simulink model "gm_parallel_8_phase_voltages"  (R2022a)
settings: Solver=FixedStepDiscrete  StartTime=0.0  StopTime=10.0  RelTol=1e-3
undefined symbols (not defined in the file or in its folder): f_c, u_dc
libraries: hdlmdlgenlib x14, simulink x2
(part 2 of 4)

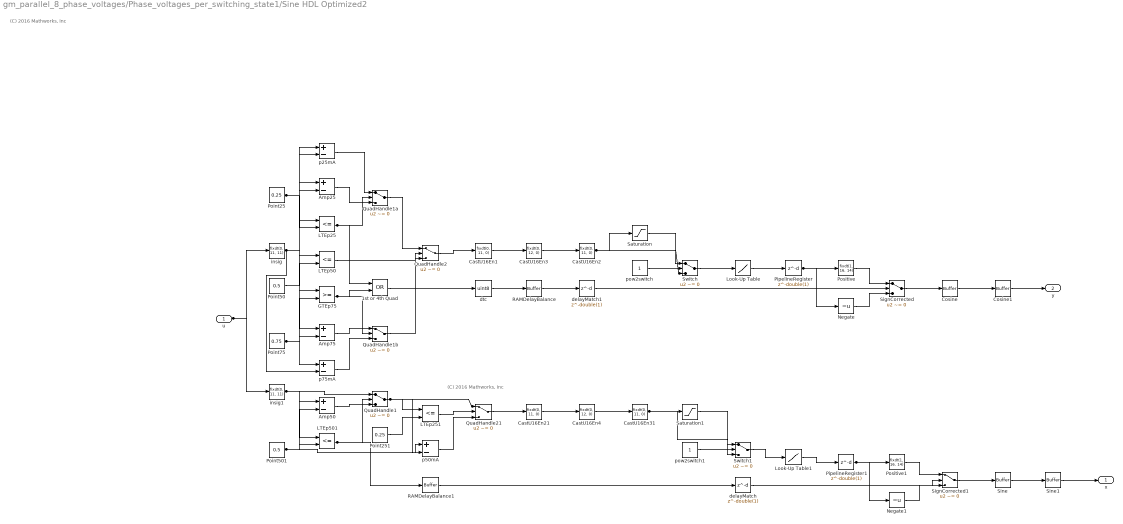
== system gm_parallel_8_phase_voltages/Phase_voltages_per_switching_state1/Sine HDL Optimized2 ==
  note: (C) 2016 Mathworks, Inc
  note: (C) 2016 Mathworks, Inc
  u : Inport  OutDataTypeStr=fixdt(1,24,20,'DataTypeOverride', 'Off')  SampleTime=1e-08
  1st or 4th Quad : Logic  Operator=OR  AllPortsSameDT=off  OutDataTypeStr=boolean  SampleTime=1e-08
  Amp25 : Sum  Inputs=+-  AccumDataTypeStr=fixdt(1, 17, 16)  OutDataTypeStr=fixdt(1, 17, 16)  SampleTime=1e-08
  Amp50 : Sum  Inputs=+-  AccumDataTypeStr=fixdt(1, 17, 16)  OutDataTypeStr=fixdt(1, 17, 16)  SampleTime=1e-08
  Amp75 : Sum  Inputs=+-  AccumDataTypeStr=fixdt(1, 17, 16)  OutDataTypeStr=fixdt(1, 17, 16)  SampleTime=1e-08
  CastU16En1 : DataTypeConversion  OutDataTypeStr=fixdt(0, 11, 0)  ConvertRealWorld=Stored Integer (SI)  SampleTime=1e-08  SaturateOnIntegerOverflow=off  RndMeth=Floor
  CastU16En2 : DataTypeConversion  OutDataTypeStr=fixdt(0, 11, 0)  ConvertRealWorld=Stored Integer (SI)  SampleTime=1e-08  RndMeth=Floor
  CastU16En21 : DataTypeConversion  OutDataTypeStr=fixdt(0, 11, 0)  ConvertRealWorld=Stored Integer (SI)  SampleTime=1e-08  SaturateOnIntegerOverflow=off  RndMeth=Floor
  CastU16En3 : DataTypeConversion  OutDataTypeStr=fixdt(0, 12, 0)  SampleTime=1e-08  SaturateOnIntegerOverflow=off  RndMeth=Floor
  CastU16En31 : DataTypeConversion  OutDataTypeStr=fixdt(0, 11, 0)  ConvertRealWorld=Stored Integer (SI)  SampleTime=1e-08  RndMeth=Floor
  CastU16En4 : DataTypeConversion  OutDataTypeStr=fixdt(0, 12, 0)  SampleTime=1e-08  SaturateOnIntegerOverflow=off  RndMeth=Floor
  Cosine : hdlmdlgenlib/Buffer
      settings: SourceProductBaseCode=SL
  Cosine1 : hdlmdlgenlib/Buffer
      settings: SourceProductBaseCode=SL
  GTEp75 : RelationalOperator  OutDataTypeStr=boolean  SampleTime=1e-08  InputSameDT=off
  LTEp{25,50,251,501} (4 alike) : RelationalOperator  Operator=<=  OutDataTypeStr=boolean  SampleTime=1e-08  InputSameDT=off
  Look-Up Table : Lookup_n-D  NumberOfTableDimensions=1  BreakpointsForDimension1="fi(\"numerictype\",numerictype(0,11,0),\"fimath\",fimath(\"RoundingMethod\", \"Floor\",\"OverflowAction\", \"Wrap\",\"ProductMode\",\"FullPrecision\",\"SumMode\",\"FullPrecision\"),\"Value\",\"[0 1 2 3 4 5 6 7 8 9 10 11 12 13 14 15 16 17 18 19 20 21 22 23 24 25 26 27 28 29 30 31 32 33 34 35 36 37 38 39 40 41 42 43 44 45 46 47 48 49 50 51 52 53 54 55 56 57 58 59 60 61 62 63 64 65 66 67 68 69 70 71 72 73 74 75 76 77 78 79 80 81 82 83 84 85 86 87 88 89 90 91 92 93 94 95 96 97 98 99 100 101 102 103 104 105 106 107 108 109 110 111 112 113 114 115 116 117 118 119 120 121 122 123 124 125 126 127 128 129 130 131 132 133 134 135 136 137 138 139 140 141 142 143 144 145 146 147 148 149 150 151 152 153 154 155 156 157 158 159 160 161 162 163 164 165 166 167 168 169 170 171 172 173 174 175 176 177 178 179 180 181 182 183 184 185 186 187 188 189 190 191 192 193 194 195 196 197 198 199 200 201 202 203 204 205 206 207 208 209 210 211 212 213 214 215 216 217 218 219 220 221 222 223 224 225 226 227 228 229 230 231 232 233 234 235 236 237 238 239 240 241 242 243 244 245 246 247 248 249 250 251 252 253 254 255 256 257 258 259 260 261 262 263 264 265 266 267 268 269 270 271 272 273 274 275 276 277 278 279 280 281 282 283 284 285 286 287 288 289 290 291 292 293 294 295 296 297 298 299 300 301 302 303 304 305 306 307 308 309 310 311 312 313 314 315 316 317 318 319 320 321 322 323 324 325 326 327 328 329 330 331 332 333 334 335 336 337 338 339 340 341 342 343 344 345 346 347 348 349 350 351 352 353 354 355 356 357 358 359 360 361 362 363 364 365 366 367 368 369 370 371 372 373 374 375 376 377 378 379 380 381 382 383 384 385 386 387 388 389 390 391 392 393 394 395 396 397 398 399 400 401 402 403 404 405 406 407 408 409 410 411 412 413 414 415 416 417 418 419 420 421 422 423 424 425 426 427 428 429 430 431 432 433 434 435 436 437 438 439 440 441 442 443 444 445 446 447 448 449 450 451 452 453 454 455 456 457 458 459 460 461 462 463 464 465 466 467 468 469 470 471 472 473 474 475 476 477 478 479 480 481 482 483 484 485 486 487 488 489 490 491 492 493 494 495 496 497 498 499 500 501 502 503 504 505 506 507 508 509 510 511]\")"  Table="reshape(fi(\"numerictype\",numerictype(1,16,14),\"fimath\",fimath(\"RoundingMethod\", \"Floor\",\"OverflowAction\", \"Wrap\",\"ProductMode\",\"FullPrecision\",\"SumMode\",\"FullPrecision\"),\"Value\",\"[0;0.0030517578125;0.00616455078125;0.00921630859375;0.01226806640625;0.015380859375;0.0184326171875;0.02154541015625;0.02459716796875;0.02764892578125;0.03076171875;0.0338134765625;0.036865234375;0.03997802734375;0.04302978515625;0.04608154296875;0.04913330078125;0.05224609375;0.0552978515625;0.058349609375;0.06146240234375;0.06451416015625;0.06756591796875;0.07061767578125;0.07373046875;0.0767822265625;0.079833984375;0.0828857421875;0.0859375;0.08905029296875;0.09210205078125;0.09515380859375;0.09820556640625;0.10125732421875;0.10430908203125;0.10736083984375;0.11041259765625;0.11346435546875;0.11651611328125;0.11956787109375;0.12261962890625;0.12567138671875;0.12872314453125;0.13177490234375;0.13482666015625;0.13787841796875;0.14093017578125;0.14398193359375;0.14703369140625;0.15008544921875;0.153076171875;0.1561279296875;0.1591796875;0.16217041015625;0.16522216796875;0.16827392578125;0.1712646484375;0.17431640625;0.1773681640625;0.18035888671875;0.18341064453125;0.1864013671875;0.189453125;0.19244384765625;0.19549560546875;0.198486328125;0.20147705078125;0.20452880859375;0.20751953125;0.21051025390625;0.2135009765625;0.216552734375;0.21954345703125;0.2225341796875;0.22552490234375;0.228515625;0.23150634765625;0.2344970703125;0.23748779296875;0.240478515625;0.24346923828125;0.24639892578125;0.2493896484375;0.25238037109375;0.25537109375;0.25830078125;0.26129150390625;0.2642822265625;0.2672119140625;0.27020263671875;0.27313232421875;0.276123046875;0.279052734375;0.281982421875;0.28497314453125;0.28790283203125;0.29083251953125;0.29376220703125;0.29669189453125;0.29962158203125;0.30255126953125;0.30548095703125;0.30841064453125;0.31134033203125;0.31427001953125;0.31719970703125;0.32012939453125;0.322998046875;0.325927734375;0.328857421875;0.33172607421875;0.33465576171875;0.3375244140625;0.34039306640625;0.34332275390625;0.34619140625;0.34906005859375;0.3519287109375;0.35479736328125;0.35772705078125;0.360595703125;0.3634033203125;0.36627197265625;0.369140625;0.37200927734375;0.3748779296875;0.377685546875;0.38055419921875;0.3834228515625;0.38623046875;0.3890380859375;0.39190673828125;0.39471435546875;0.39752197265625;0.400390625;0.4031982421875;0.406005859375;0.4088134765625;0.41162109375;0.41436767578125;0.41717529296875;0.41998291015625;0.42279052734375;0.425537109375;0.4283447265625;0.43109130859375;0.43389892578125;0.4366455078125;0.43939208984375;0.44219970703125;0.4449462890625;0.44769287109375;0.450439453125;0.45318603515625;0.4559326171875;0.4586181640625;0.46136474609375;0.464111328125;0.466796875;0.46954345703125;0.47222900390625;0.4749755859375;0.4776611328125;0.4803466796875;0.4830322265625;0.4857177734375;0.4884033203125;0.4910888671875;0.4937744140625;0.4964599609375;0.49908447265625;0.50177001953125;0.50445556640625;0.507080078125;0.50970458984375;0.51239013671875;0.5150146484375;0.51763916015625;0.520263671875;0.52288818359375;0.5255126953125;0.52813720703125;0.53070068359375;0.5333251953125;0.53594970703125;0.53851318359375;0.5411376953125;0.543701171875;0.5462646484375;0.548828125;0.5513916015625;0.553955078125;0.5565185546875;0.55908203125;0.5616455078125;0.56414794921875;0.56671142578125;0.5692138671875;0.57177734375;0.57427978515625;0.5767822265625;0.57928466796875;0.581787109375;0.58428955078125;0.5867919921875;0.58929443359375;0.59173583984375;0.59423828125;0.5966796875;0.59918212890625;0.60162353515625;0.60406494140625;0.60650634765625;0.60894775390625;0.61138916015625;0.61383056640625;0.61627197265625;0.61865234375;0.62109375;0.62347412109375;0.62591552734375;0.6282958984375;0.63067626953125;0.633056640625;0.63543701171875;0.6378173828125;0.64019775390625;0.64251708984375;0.6448974609375;0.647216796875;0.6495361328125;0.65191650390625;0.65423583984375;0.65655517578125;0.65887451171875;0.66119384765625;0.6634521484375;0.665771484375;0.6680908203125;0.67034912109375;0.672607421875;0.6749267578125;0.67718505859375;0.679443359375;0.68170166015625;0.68389892578125;0.6861572265625;0.68841552734375 ...(+4183 chars)]\"), [1  512])"  InterpMethod=Flat  ExtrapMethod=Clip  DiagnosticForOutOfRangeInput=Error  SampleTime=1e-08  OutDataTypeStr=fixdt(1, 16, 14)
  Look-Up Table1 : Lookup_n-D  NumberOfTableDimensions=1  BreakpointsForDimension1="fi(\"numerictype\",numerictype(0,11,0),\"fimath\",fimath(\"RoundingMethod\", \"Floor\",\"OverflowAction\", \"Wrap\",\"ProductMode\",\"FullPrecision\",\"SumMode\",\"FullPrecision\"),\"Value\",\"[0 1 2 3 4 5 6 7 8 9 10 11 12 13 14 15 16 17 18 19 20 21 22 23 24 25 26 27 28 29 30 31 32 33 34 35 36 37 38 39 40 41 42 43 44 45 46 47 48 49 50 51 52 53 54 55 56 57 58 59 60 61 62 63 64 65 66 67 68 69 70 71 72 73 74 75 76 77 78 79 80 81 82 83 84 85 86 87 88 89 90 91 92 93 94 95 96 97 98 99 100 101 102 103 104 105 106 107 108 109 110 111 112 113 114 115 116 117 118 119 120 121 122 123 124 125 126 127 128 129 130 131 132 133 134 135 136 137 138 139 140 141 142 143 144 145 146 147 148 149 150 151 152 153 154 155 156 157 158 159 160 161 162 163 164 165 166 167 168 169 170 171 172 173 174 175 176 177 178 179 180 181 182 183 184 185 186 187 188 189 190 191 192 193 194 195 196 197 198 199 200 201 202 203 204 205 206 207 208 209 210 211 212 213 214 215 216 217 218 219 220 221 222 223 224 225 226 227 228 229 230 231 232 233 234 235 236 237 238 239 240 241 242 243 244 245 246 247 248 249 250 251 252 253 254 255 256 257 258 259 260 261 262 263 264 265 266 267 268 269 270 271 272 273 274 275 276 277 278 279 280 281 282 283 284 285 286 287 288 289 290 291 292 293 294 295 296 297 298 299 300 301 302 303 304 305 306 307 308 309 310 311 312 313 314 315 316 317 318 319 320 321 322 323 324 325 326 327 328 329 330 331 332 333 334 335 336 337 338 339 340 341 342 343 344 345 346 347 348 349 350 351 352 353 354 355 356 357 358 359 360 361 362 363 364 365 366 367 368 369 370 371 372 373 374 375 376 377 378 379 380 381 382 383 384 385 386 387 388 389 390 391 392 393 394 395 396 397 398 399 400 401 402 403 404 405 406 407 408 409 410 411 412 413 414 415 416 417 418 419 420 421 422 423 424 425 426 427 428 429 430 431 432 433 434 435 436 437 438 439 440 441 442 443 444 445 446 447 448 449 450 451 452 453 454 455 456 457 458 459 460 461 462 463 464 465 466 467 468 469 470 471 472 473 474 475 476 477 478 479 480 481 482 483 484 485 486 487 488 489 490 491 492 493 494 495 496 497 498 499 500 501 502 503 504 505 506 507 508 509 510 511]\")"  Table="reshape(fi(\"numerictype\",numerictype(1,16,14),\"fimath\",fimath(\"RoundingMethod\", \"Floor\",\"OverflowAction\", \"Wrap\",\"ProductMode\",\"FullPrecision\",\"SumMode\",\"FullPrecision\"),\"Value\",\"[0;0.0030517578125;0.00616455078125;0.00921630859375;0.01226806640625;0.015380859375;0.0184326171875;0.02154541015625;0.02459716796875;0.02764892578125;0.03076171875;0.0338134765625;0.036865234375;0.03997802734375;0.04302978515625;0.04608154296875;0.04913330078125;0.05224609375;0.0552978515625;0.058349609375;0.06146240234375;0.06451416015625;0.06756591796875;0.07061767578125;0.07373046875;0.0767822265625;0.079833984375;0.0828857421875;0.0859375;0.08905029296875;0.09210205078125;0.09515380859375;0.09820556640625;0.10125732421875;0.10430908203125;0.10736083984375;0.11041259765625;0.11346435546875;0.11651611328125;0.11956787109375;0.12261962890625;0.12567138671875;0.12872314453125;0.13177490234375;0.13482666015625;0.13787841796875;0.14093017578125;0.14398193359375;0.14703369140625;0.15008544921875;0.153076171875;0.1561279296875;0.1591796875;0.16217041015625;0.16522216796875;0.16827392578125;0.1712646484375;0.17431640625;0.1773681640625;0.18035888671875;0.18341064453125;0.1864013671875;0.189453125;0.19244384765625;0.19549560546875;0.198486328125;0.20147705078125;0.20452880859375;0.20751953125;0.21051025390625;0.2135009765625;0.216552734375;0.21954345703125;0.2225341796875;0.22552490234375;0.228515625;0.23150634765625;0.2344970703125;0.23748779296875;0.240478515625;0.24346923828125;0.24639892578125;0.2493896484375;0.25238037109375;0.25537109375;0.25830078125;0.26129150390625;0.2642822265625;0.2672119140625;0.27020263671875;0.27313232421875;0.276123046875;0.279052734375;0.281982421875;0.28497314453125;0.28790283203125;0.29083251953125;0.29376220703125;0.29669189453125;0.29962158203125;0.30255126953125;0.30548095703125;0.30841064453125;0.31134033203125;0.31427001953125;0.31719970703125;0.32012939453125;0.322998046875;0.325927734375;0.328857421875;0.33172607421875;0.33465576171875;0.3375244140625;0.34039306640625;0.34332275390625;0.34619140625;0.34906005859375;0.3519287109375;0.35479736328125;0.35772705078125;0.360595703125;0.3634033203125;0.36627197265625;0.369140625;0.37200927734375;0.3748779296875;0.377685546875;0.38055419921875;0.3834228515625;0.38623046875;0.3890380859375;0.39190673828125;0.39471435546875;0.39752197265625;0.400390625;0.4031982421875;0.406005859375;0.4088134765625;0.41162109375;0.41436767578125;0.41717529296875;0.41998291015625;0.42279052734375;0.425537109375;0.4283447265625;0.43109130859375;0.43389892578125;0.4366455078125;0.43939208984375;0.44219970703125;0.4449462890625;0.44769287109375;0.450439453125;0.45318603515625;0.4559326171875;0.4586181640625;0.46136474609375;0.464111328125;0.466796875;0.46954345703125;0.47222900390625;0.4749755859375;0.4776611328125;0.4803466796875;0.4830322265625;0.4857177734375;0.4884033203125;0.4910888671875;0.4937744140625;0.4964599609375;0.49908447265625;0.50177001953125;0.50445556640625;0.507080078125;0.50970458984375;0.51239013671875;0.5150146484375;0.51763916015625;0.520263671875;0.52288818359375;0.5255126953125;0.52813720703125;0.53070068359375;0.5333251953125;0.53594970703125;0.53851318359375;0.5411376953125;0.543701171875;0.5462646484375;0.548828125;0.5513916015625;0.553955078125;0.5565185546875;0.55908203125;0.5616455078125;0.56414794921875;0.56671142578125;0.5692138671875;0.57177734375;0.57427978515625;0.5767822265625;0.57928466796875;0.581787109375;0.58428955078125;0.5867919921875;0.58929443359375;0.59173583984375;0.59423828125;0.5966796875;0.59918212890625;0.60162353515625;0.60406494140625;0.60650634765625;0.60894775390625;0.61138916015625;0.61383056640625;0.61627197265625;0.61865234375;0.62109375;0.62347412109375;0.62591552734375;0.6282958984375;0.63067626953125;0.633056640625;0.63543701171875;0.6378173828125;0.64019775390625;0.64251708984375;0.6448974609375;0.647216796875;0.6495361328125;0.65191650390625;0.65423583984375;0.65655517578125;0.65887451171875;0.66119384765625;0.6634521484375;0.665771484375;0.6680908203125;0.67034912109375;0.672607421875;0.6749267578125;0.67718505859375;0.679443359375;0.68170166015625;0.68389892578125;0.6861572265625;0.68841552734375 ...(+4183 chars)]\"), [1  512])"  InterpMethod=Flat  ExtrapMethod=Clip  DiagnosticForOutOfRangeInput=Error  SampleTime=1e-08  OutDataTypeStr=fixdt(1, 16, 14)
  Negate : UnaryMinus  SampleTime=1e-08
  Negate1 : UnaryMinus  SampleTime=1e-08
  PipelineRegister : Delay  DelayLength=double(1)  InitialCondition=0  SampleTime=1e-08
  PipelineRegister1 : Delay  DelayLength=double(1)  InitialCondition=0  SampleTime=1e-08
  Point25 : Constant  Value=0.25  OutDataTypeStr=fixdt(0, 16, 16)  SampleTime=1e-08
  Point251 : Constant  Value=0.25  OutDataTypeStr=fixdt(0, 16, 16)  SampleTime=1e-08
  Point50 : Constant  Value=0.5  OutDataTypeStr=fixdt(0, 16, 16)  SampleTime=1e-08
  Point501 : Constant  Value=0.5  OutDataTypeStr=fixdt(0, 16, 16)  SampleTime=1e-08
  Point75 : Constant  Value=0.75  OutDataTypeStr=fixdt(0, 16, 16)  SampleTime=1e-08
  Positive : DataTypeConversion  OutDataTypeStr=fixdt(1, 16, 14)  SampleTime=1e-08  SaturateOnIntegerOverflow=off  RndMeth=Floor
  Positive1 : DataTypeConversion  OutDataTypeStr=fixdt(1, 16, 14)  SampleTime=1e-08  SaturateOnIntegerOverflow=off  RndMeth=Floor
  QuadHandle1 : Switch  Criteria=u2 ~= 0  Threshold=double(0)  OutDataTypeStr=fixdt(1, 17, 16)  SampleTime=1e-08  SaturateOnIntegerOverflow=off  InputSameDT=off
  QuadHandle1a : Switch  Criteria=u2 ~= 0  Threshold=double(0)  OutDataTypeStr=fixdt(1, 17, 16)  SampleTime=1e-08  SaturateOnIntegerOverflow=off  InputSameDT=off
  QuadHandle1b : Switch  Criteria=u2 ~= 0  Threshold=double(0)  OutDataTypeStr=fixdt(1, 17, 16)  SampleTime=1e-08  SaturateOnIntegerOverflow=off  InputSameDT=off
  QuadHandle2 : Switch  Criteria=u2 ~= 0  Threshold=double(0)  OutDataTypeStr=fixdt(0, 11, 11)  SampleTime=1e-08  InputSameDT=off
  QuadHandle21 : Switch  Criteria=u2 ~= 0  Threshold=double(0)  OutDataTypeStr=fixdt(0, 11, 11)  SampleTime=1e-08  SaturateOnIntegerOverflow=off  InputSameDT=off
  RAMDelayBalance : hdlmdlgenlib/Buffer
      settings: SourceProductBaseCode=SL
  RAMDelayBalance1 : hdlmdlgenlib/Buffer
      settings: SourceProductBaseCode=SL
  Saturation : Saturate  UpperLimit="fi(0,0,11,0,\"hex\",\"1ff\")"  LowerLimit="fi(0,0,11,0,\"hex\",\"000\")"  SampleTime=1e-08  OutDataTypeStr=fixdt(0, 11, 0)
  Saturation1 : Saturate  UpperLimit="fi(0,0,11,0,\"hex\",\"1ff\")"  LowerLimit="fi(0,0,11,0,\"hex\",\"000\")"  SampleTime=1e-08  OutDataTypeStr=fixdt(0, 11, 0)
  SignCorrected : Switch  Criteria=u2 ~= 0  Threshold=double(0)  OutDataTypeStr=fixdt(1, 16, 14)  SampleTime=1e-08  SaturateOnIntegerOverflow=off  InputSameDT=off
  SignCorrected1 : Switch  Criteria=u2 ~= 0  Threshold=double(0)  OutDataTypeStr=fixdt(1, 16, 14)  SampleTime=1e-08  SaturateOnIntegerOverflow=off  InputSameDT=off
  Sine : hdlmdlgenlib/Buffer
      settings: SourceProductBaseCode=SL
  Sine1 : hdlmdlgenlib/Buffer
      settings: SourceProductBaseCode=SL
  Switch : Switch  Criteria=u2 ~= 0  Threshold=double(0)  OutDataTypeStr=fixdt(0, 11, 0)  SampleTime=1e-08  SaturateOnIntegerOverflow=off  InputSameDT=off
  Switch1 : Switch  Criteria=u2 ~= 0  Threshold=double(0)  OutDataTypeStr=fixdt(0, 11, 0)  SampleTime=1e-08  SaturateOnIntegerOverflow=off  InputSameDT=off
  delayMatch : Delay  DelayLength=double(1)  InitialCondition=0  SampleTime=1e-08
  delayMatch1 : Delay  DelayLength=double(1)  InitialCondition=0  SampleTime=1e-08
  dtc : DataTypeConversion  OutDataTypeStr=uint8  SampleTime=1e-08  SaturateOnIntegerOverflow=off  RndMeth=Floor
  insig : DataTypeConversion  OutDataTypeStr=fixdt(0, 11, 11)  SampleTime=1e-08  SaturateOnIntegerOverflow=off  RndMeth=Floor
  insig1 : DataTypeConversion  OutDataTypeStr=fixdt(0, 11, 11)  SampleTime=1e-08  SaturateOnIntegerOverflow=off  RndMeth=Floor
  p25mA : Sum  Inputs=+-  AccumDataTypeStr=fixdt(1, 17, 16)  OutDataTypeStr=fixdt(1, 17, 16)  SampleTime=1e-08
  p50mA : Sum  Inputs=+-  AccumDataTypeStr=fixdt(1, 18, 16)  OutDataTypeStr=fixdt(1, 18, 16)  SampleTime=1e-08
  p75mA : Sum  Inputs=+-  AccumDataTypeStr=fixdt(1, 17, 16)  OutDataTypeStr=fixdt(1, 17, 16)  SampleTime=1e-08
  pow2switch : Constant  OutDataTypeStr=boolean  SampleTime=1e-08
  pow2switch1 : Constant  OutDataTypeStr=boolean  SampleTime=1e-08
  x : Outport  SampleTime=1e-08
  y : Outport  Port=2  SampleTime=1e-08
  wires:
  Sine1/1 -> x/1
  Cosine1/1 -> y/1
  Cosine/1 -> Cosine1/1
  Sine/1 -> Sine1/1
  dtc/1 -> RAMDelayBalance/1
  Amp25/1 -> QuadHandle1a/3
  Amp75/1 -> QuadHandle1b/1
  CastU16En1/1 -> CastU16En3/1
  CastU16En2/1 -> Switch/3, Saturation/1
  CastU16En3/1 -> CastU16En2/1
  GTEp75/1 -> QuadHandle1b/2, 1st or 4th Quad/2
  LTEp25/1 -> QuadHandle1a/2, 1st or 4th Quad/1
  LTEp50/1 -> QuadHandle2/2
  PipelineRegister/1 -> Positive/1, Negate/1
  Negate/1 -> SignCorrected/3
  Point25/1 -> p25mA/1, LTEp25/2, Amp25/2
  Point50/1 -> LTEp50/2
  Point75/1 -> p75mA/1, GTEp75/2, Amp75/2
  Positive/1 -> SignCorrected/1
  QuadHandle1a/1 -> QuadHandle2/1
  QuadHandle1b/1 -> QuadHandle2/3
  QuadHandle2/1 -> CastU16En1/1
  delayMatch1/1 -> SignCorrected/2
  Saturation/1 -> Switch/1
  SignCorrected/1 -> Cosine/1
  Switch/1 -> Look-Up Table/1
  insig/1 -> p75mA/2, p25mA/2, LTEp50/1, LTEp25/1, GTEp75/1, Amp75/1, Amp25/1
  p25mA/1 -> QuadHandle1a/1
  p75mA/1 -> QuadHandle1b/3
  pow2switch/1 -> Switch/2
  Amp50/1 -> QuadHandle1/3
  CastU16En21/1 -> CastU16En4/1
  CastU16En31/1 -> Switch1/3, Saturation1/1
  CastU16En4/1 -> CastU16En31/1
  LTEp251/1 -> QuadHandle21/2
  LTEp501/1 -> QuadHandle1/2, RAMDelayBalance1/1
  PipelineRegister1/1 -> Positive1/1, Negate1/1
  Negate1/1 -> SignCorrected1/3
  Point251/1 -> LTEp251/2
  Point501/1 -> p50mA/1, LTEp501/2, Amp50/2
  Positive1/1 -> SignCorrected1/1
  QuadHandle1/1 -> p50mA/2, QuadHandle21/1, LTEp251/1
  QuadHandle21/1 -> CastU16En21/1
  delayMatch/1 -> SignCorrected1/2
  Saturation1/1 -> Switch1/1
  SignCorrected1/1 -> Sine/1
  Switch1/1 -> Look-Up Table1/1
  insig1/1 -> QuadHandle1/1, LTEp501/1, Amp50/1
  p50mA/1 -> QuadHandle21/3
  pow2switch1/1 -> Switch1/2
  1st or 4th Quad/1 -> dtc/1
  RAMDelayBalance1/1 -> delayMatch/1
  RAMDelayBalance/1 -> delayMatch1/1
  u/1 -> insig1/1, insig/1
  Look-Up Table/1 -> PipelineRegister/1
  Look-Up Table1/1 -> PipelineRegister1/1

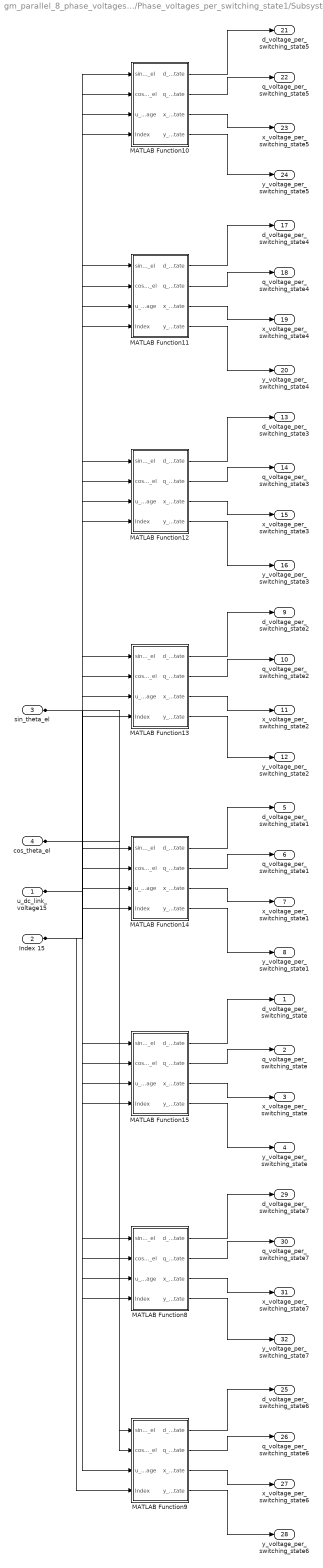
== system gm_parallel_8_phase_voltages/Phase_voltages_per_switching_state1/Subsystem ==
  u_dc_link_voltage15 : Inport  OutDataTypeStr=single  PortDimensions=1  SampleTime=1e-08
  Index 15 : Inport  Port=2  OutDataTypeStr=int32  PortDimensions=1  SampleTime=1e-08
  sin_theta_el : Inport  Port=3  OutDataTypeStr=single  PortDimensions=1  SampleTime=1e-08
  cos_theta_el : Inport  Port=4  OutDataTypeStr=single  PortDimensions=1  SampleTime=1e-08
  MATLAB Function10 : Subsystem
  MATLAB Function11 : Subsystem
  MATLAB Function12 : Subsystem
  MATLAB Function13 : Subsystem
  MATLAB Function14 : Subsystem
  MATLAB Function15 : Subsystem
  MATLAB Function8 : Subsystem
  MATLAB Function9 : Subsystem
  d_voltage_per_switching_state : Outport  SampleTime=1e-08
  q_voltage_per_switching_state : Outport  Port=2  SampleTime=1e-08
  x_voltage_per_switching_state : Outport  Port=3  SampleTime=1e-08
  y_voltage_per_switching_state : Outport  Port=4  SampleTime=1e-08
  d_voltage_per_switching_state1 : Outport  Port=5  SampleTime=1e-08
  q_voltage_per_switching_state1 : Outport  Port=6  SampleTime=1e-08
  x_voltage_per_switching_state1 : Outport  Port=7  SampleTime=1e-08
  y_voltage_per_switching_state1 : Outport  Port=8  SampleTime=1e-08
  d_voltage_per_switching_state2 : Outport  Port=9  SampleTime=1e-08
  q_voltage_per_switching_state2 : Outport  Port=10  SampleTime=1e-08
  x_voltage_per_switching_state2 : Outport  Port=11  SampleTime=1e-08
  y_voltage_per_switching_state2 : Outport  Port=12  SampleTime=1e-08
  d_voltage_per_switching_state3 : Outport  Port=13  SampleTime=1e-08
  q_voltage_per_switching_state3 : Outport  Port=14  SampleTime=1e-08
  x_voltage_per_switching_state3 : Outport  Port=15  SampleTime=1e-08
  y_voltage_per_switching_state3 : Outport  Port=16  SampleTime=1e-08
  d_voltage_per_switching_state4 : Outport  Port=17  SampleTime=1e-08
  q_voltage_per_switching_state4 : Outport  Port=18  SampleTime=1e-08
  x_voltage_per_switching_state4 : Outport  Port=19  SampleTime=1e-08
  y_voltage_per_switching_state4 : Outport  Port=20  SampleTime=1e-08
  d_voltage_per_switching_state5 : Outport  Port=21  SampleTime=1e-08
  q_voltage_per_switching_state5 : Outport  Port=22  SampleTime=1e-08
  x_voltage_per_switching_state5 : Outport  Port=23  SampleTime=1e-08
  y_voltage_per_switching_state5 : Outport  Port=24  SampleTime=1e-08
  d_voltage_per_switching_state6 : Outport  Port=25  SampleTime=1e-08
  q_voltage_per_switching_state6 : Outport  Port=26  SampleTime=1e-08
  x_voltage_per_switching_state6 : Outport  Port=27  SampleTime=1e-08
  y_voltage_per_switching_state6 : Outport  Port=28  SampleTime=1e-08
  d_voltage_per_switching_state7 : Outport  Port=29  SampleTime=1e-08
  q_voltage_per_switching_state7 : Outport  Port=30  SampleTime=1e-08
  x_voltage_per_switching_state7 : Outport  Port=31  SampleTime=1e-08
  y_voltage_per_switching_state7 : Outport  Port=32  SampleTime=1e-08
  wires:
  MATLAB Function10/1(d_voltage_per_switching_state) -> d_voltage_per_switching_state5/1
  MATLAB Function10/2(q_voltage_per_switching_state) -> q_voltage_per_switching_state5/1
  MATLAB Function10/3(x_voltage_per_switching_state) -> x_voltage_per_switching_state5/1
  MATLAB Function10/4(y_voltage_per_switching_state) -> y_voltage_per_switching_state5/1
  MATLAB Function11/1(d_voltage_per_switching_state) -> d_voltage_per_switching_state4/1
  MATLAB Function11/2(q_voltage_per_switching_state) -> q_voltage_per_switching_state4/1
  MATLAB Function11/3(x_voltage_per_switching_state) -> x_voltage_per_switching_state4/1
  MATLAB Function11/4(y_voltage_per_switching_state) -> y_voltage_per_switching_state4/1
  MATLAB Function12/1(d_voltage_per_switching_state) -> d_voltage_per_switching_state3/1
  MATLAB Function12/2(q_voltage_per_switching_state) -> q_voltage_per_switching_state3/1
  MATLAB Function12/3(x_voltage_per_switching_state) -> x_voltage_per_switching_state3/1
  MATLAB Function12/4(y_voltage_per_switching_state) -> y_voltage_per_switching_state3/1
  MATLAB Function13/1(d_voltage_per_switching_state) -> d_voltage_per_switching_state2/1
  MATLAB Function13/2(q_voltage_per_switching_state) -> q_voltage_per_switching_state2/1
  MATLAB Function13/3(x_voltage_per_switching_state) -> x_voltage_per_switching_state2/1
  MATLAB Function13/4(y_voltage_per_switching_state) -> y_voltage_per_switching_state2/1
  MATLAB Function14/1(d_voltage_per_switching_state) -> d_voltage_per_switching_state1/1
  MATLAB Function14/2(q_voltage_per_switching_state) -> q_voltage_per_switching_state1/1
  MATLAB Function14/3(x_voltage_per_switching_state) -> x_voltage_per_switching_state1/1
  MATLAB Function14/4(y_voltage_per_switching_state) -> y_voltage_per_switching_state1/1
  MATLAB Function15/1(d_voltage_per_switching_state) -> d_voltage_per_switching_state/1
  MATLAB Function15/2(q_voltage_per_switching_state) -> q_voltage_per_switching_state/1
  MATLAB Function15/3(x_voltage_per_switching_state) -> x_voltage_per_switching_state/1
  MATLAB Function15/4(y_voltage_per_switching_state) -> y_voltage_per_switching_state/1
  MATLAB Function8/1(d_voltage_per_switching_state) -> d_voltage_per_switching_state7/1
  MATLAB Function8/2(q_voltage_per_switching_state) -> q_voltage_per_switching_state7/1
  MATLAB Function8/3(x_voltage_per_switching_state) -> x_voltage_per_switching_state7/1
  MATLAB Function8/4(y_voltage_per_switching_state) -> y_voltage_per_switching_state7/1
  MATLAB Function9/1(d_voltage_per_switching_state) -> d_voltage_per_switching_state6/1
  MATLAB Function9/2(q_voltage_per_switching_state) -> q_voltage_per_switching_state6/1
  MATLAB Function9/3(x_voltage_per_switching_state) -> x_voltage_per_switching_state6/1
  MATLAB Function9/4(y_voltage_per_switching_state) -> y_voltage_per_switching_state6/1
  u_dc_link_voltage15/1 -> MATLAB Function9/3(u_dc_link_voltage), MATLAB Function8/3(u_dc_link_voltage), MATLAB Function15/3(u_dc_link_voltage), MATLAB Function14/3(u_dc_link_voltage), MATLAB Function13/3(u_dc_link_voltage), MATLAB Function12/3(u_dc_link_voltage), MATLAB Function11/3(u_dc_link_voltage), MATLAB Function10/3(u_dc_link_voltage)
  Index 15/1 -> MATLAB Function9/4(Index), MATLAB Function8/4(Index), MATLAB Function15/4(Index), MATLAB Function14/4(Index), MATLAB Function13/4(Index), MATLAB Function12/4(Index), MATLAB Function11/4(Index), MATLAB Function10/4(Index)
  sin_theta_el/1 -> MATLAB Function9/1(sin_theta_el), MATLAB Function8/1(sin_theta_el), MATLAB Function15/1(sin_theta_el), MATLAB Function14/1(sin_theta_el), MATLAB Function13/1(sin_theta_el), MATLAB Function12/1(sin_theta_el), MATLAB Function11/1(sin_theta_el), MATLAB Function10/1(sin_theta_el)
  cos_theta_el/1 -> MATLAB Function9/2(cos_theta_el), MATLAB Function8/2(cos_theta_el), MATLAB Function15/2(cos_theta_el), MATLAB Function14/2(cos_theta_el), MATLAB Function13/2(cos_theta_el), MATLAB Function12/2(cos_theta_el), MATLAB Function11/2(cos_theta_el), MATLAB Function10/2(cos_theta_el)

== system gm_parallel_8_phase_voltages/Phase_voltages_per_switching_state1/Detect Rise Positive/Positive ==
  u : Inport  OutDataTypeStr=boolean  SampleTime=1e-08
  Compare : RelationalOperator  Operator=>  OutDataTypeStr=boolean  ZeroCross=off
  Constant : Constant  DisableCoverage=on  Value=0  OutDataTypeStr=Inherit: Inherit via back propagation  SampleTime=-1  PreserveConstantTs=on
  y : Outport  SampleTime=1e-08
  wires:
  Compare/1 -> y/1
  Constant/1 -> Compare/2
  u/1 -> Compare/1

== system gm_parallel_8_phase_voltages/Phase_voltages_per_switching_state1/Detect Rise Positive2/Positive ==
  u : Inport  OutDataTypeStr=boolean  SampleTime=1e-08
  Compare : RelationalOperator  Operator=>  OutDataTypeStr=boolean  ZeroCross=off
  Constant : Constant  DisableCoverage=on  Value=0  OutDataTypeStr=Inherit: Inherit via back propagation  SampleTime=-1  PreserveConstantTs=on
  y : Outport  SampleTime=1e-08
  wires:
  Compare/1 -> y/1
  Constant/1 -> Compare/2
  u/1 -> Compare/1

== system gm_parallel_8_phase_voltages/Phase_voltages_per_switching_state1/Detect Rise Positive3/Positive ==
  u : Inport  OutDataTypeStr=boolean  SampleTime=1e-08
  Compare : RelationalOperator  Operator=>  OutDataTypeStr=boolean  ZeroCross=off
  Constant : Constant  DisableCoverage=on  Value=0  OutDataTypeStr=Inherit: Inherit via back propagation  SampleTime=-1  PreserveConstantTs=on
  y : Outport  SampleTime=1e-08
  wires:
  Compare/1 -> y/1
  Constant/1 -> Compare/2
  u/1 -> Compare/1

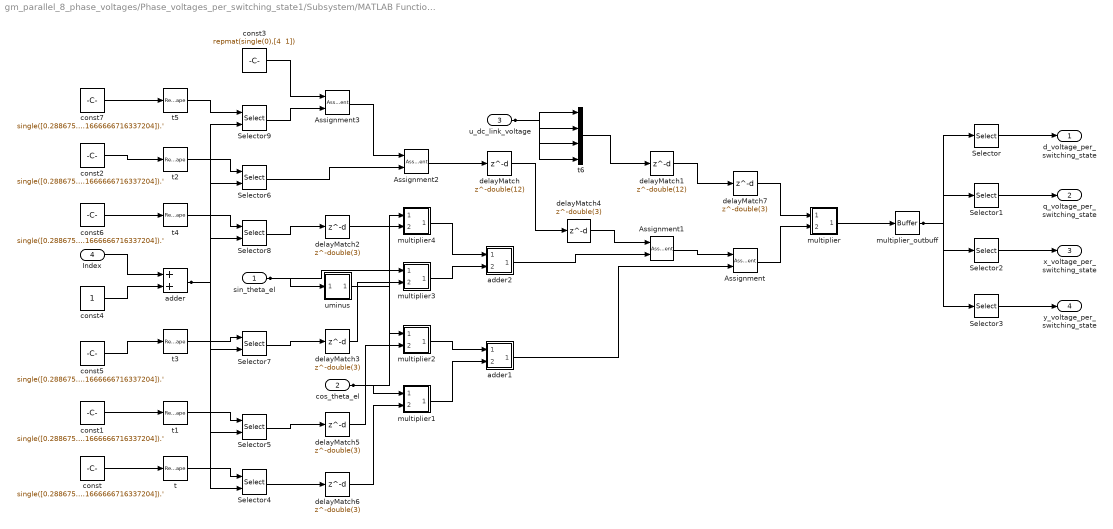
== system gm_parallel_8_phase_voltages/Phase_voltages_per_switching_state1/Subsystem/MATLAB Function10 ==
  sin_theta_el : Inport  OutDataTypeStr=single  PortDimensions=1  SampleTime=1e-08
  cos_theta_el : Inport  Port=2  OutDataTypeStr=single  PortDimensions=1  SampleTime=1e-08
  u_dc_link_voltage : Inport  Port=3  OutDataTypeStr=single  PortDimensions=1  SampleTime=1e-08
  Index : Inport  Port=4  OutDataTypeStr=int32  PortDimensions=1  SampleTime=1e-08
  Assignment : Assignment  NumberOfDimensions=2  SampleTime=1e-08  IndexOptions=Index vector (dialog),Index vector (dialog)  Indices=double(2),double(1)  OutputSizes=double(0),double(0)
  Assignment1 : Assignment  NumberOfDimensions=2  SampleTime=1e-08  IndexOptions=Index vector (dialog),Index vector (dialog)  Indices=double(1),double(1)  OutputSizes=double(0),double(0)
  Assignment2 : Assignment  NumberOfDimensions=2  SampleTime=1e-08  IndexOptions=Index vector (dialog),Index vector (dialog)  Indices=double(4),double(1)  OutputSizes=double(0),double(0)
  Assignment3 : Assignment  NumberOfDimensions=2  SampleTime=1e-08  IndexOptions=Index vector (dialog),Index vector (dialog)  Indices=double(3),double(1)  OutputSizes=double(0),double(0)
  Selector : Selector  NumberOfDimensions=2  SampleTime=1e-08  IndexOptions=Index vector (dialog),Index vector (dialog)  Indices=double(1),double(1)  OutputSizes=double(0),double(0)
  Selector1 : Selector  NumberOfDimensions=2  SampleTime=1e-08  IndexOptions=Index vector (dialog),Index vector (dialog)  Indices=double(2),double(1)  OutputSizes=double(0),double(0)
  Selector2 : Selector  NumberOfDimensions=2  SampleTime=1e-08  IndexOptions=Index vector (dialog),Index vector (dialog)  Indices=double(3),double(1)  OutputSizes=double(0),double(0)
  Selector3 : Selector  NumberOfDimensions=2  SampleTime=1e-08  IndexOptions=Index vector (dialog),Index vector (dialog)  Indices=double(4),double(1)  OutputSizes=double(0),double(0)
  Selector4 : Selector  NumberOfDimensions=2  SampleTime=1e-08  IndexOptions=Index vector (dialog),Index vector (port)  Indices=double(2),double(-1)  OutputSizes=double(0),double(0)
  Selector5 : Selector  NumberOfDimensions=2  SampleTime=1e-08  IndexOptions=Index vector (dialog),Index vector (port)  Indices=double(1),double(-1)  OutputSizes=double(0),double(0)
  Selector6 : Selector  NumberOfDimensions=2  SampleTime=1e-08  IndexOptions=Index vector (dialog),Index vector (port)  Indices=double(4),double(-1)  OutputSizes=double(0),double(0)
  Selector7 : Selector  NumberOfDimensions=2  SampleTime=1e-08  IndexOptions=Index vector (dialog),Index vector (port)  Indices=double(2),double(-1)  OutputSizes=double(0),double(0)
  Selector8 : Selector  NumberOfDimensions=2  SampleTime=1e-08  IndexOptions=Index vector (dialog),Index vector (port)  Indices=double(1),double(-1)  OutputSizes=double(0),double(0)
  Selector9 : Selector  NumberOfDimensions=2  SampleTime=1e-08  IndexOptions=Index vector (dialog),Index vector (port)  Indices=double(3),double(-1)  OutputSizes=double(0),double(0)
  adder : Sum  AccumDataTypeStr=int32  OutDataTypeStr=int32  RndMeth=Nearest  SaturateOnIntegerOverflow=on  SampleTime=1e-08
  adder1 : Subsystem
      mask Display: disp('NFP\nadd');
  adder2 : Subsystem
      mask Display: disp('NFP\nadd');
  const{,1..2,5..7} (6 alike) : Constant  Value=single([0.28867512941360474 -0.1666666716337204 -0.28867512941360474 -0.1666666716337204 0.6220084428787231 -0.1666666716337204 0.044658198952674866 -0.1666666716337204 0.12200846523046494 0.12200846523046494 -0.45534181594848633 -0.45534181594848633 0.45534181594848633 0.12200846523046494 -0.12200846523046494 -0.45534181594848633 0.12200846523046494 -0.45534181594848633 -0.45534181594848633 0.12200846523046494 0.45534181594848633 -0.45534181594848633 -0.12200846523046494 0.12200846523046494 -0.044658198952674866 -0.1666666716337204 -0.6220084428787231 -0.1666666716337204 0.28867512941360474 -0.1666666716337204 -0.28867512941360474 -0.1666666716337204]).'  VectorParams1D=off  OutDataTypeStr=single  SampleTime=1e-08
  const3 : Constant  Value="repmat(single(0),[4  1])"  VectorParams1D=off  OutDataTypeStr=single  SampleTime=1e-08
  const4 : Constant  VectorParams1D=off  OutDataTypeStr=int32  SampleTime=1e-08
  delayMatch : Delay  DelayLength=double(12)  InitialCondition=0  SampleTime=1e-08
  delayMatch1 : Delay  DelayLength=double(12)  InitialCondition=0  SampleTime=1e-08
  delayMatch{2..7} (6 alike) : Delay  DelayLength=double(3)  InitialCondition=0  SampleTime=1e-08
  multiplier : Subsystem
      mask Display: disp('NFP\nmul');
  multiplier1 : Subsystem
      mask Display: disp('NFP\nmul');
  multiplier2 : Subsystem
      mask Display: disp('NFP\nmul');
  multiplier3 : Subsystem
      mask Display: disp('NFP\nmul');
  multiplier4 : Subsystem
      mask Display: disp('NFP\nmul');
  multiplier_outbuff : hdlmdlgenlib/Buffer
      settings: SourceProductBaseCode=SL
  t{,1..5} (6 alike) : Reshape  OutputDimensionality=Customize  OutputDimensions=[4,8]
  t6 : Mux
  uminus : Subsystem
      mask Display: disp('NFP\numinus');
  d_voltage_per_switching_state : Outport  SampleTime=1e-08  VectorParamsAs1DForOutWhenUnconnected=off
  q_voltage_per_switching_state : Outport  Port=2  SampleTime=1e-08
  x_voltage_per_switching_state : Outport  Port=3  SampleTime=1e-08
  y_voltage_per_switching_state : Outport  Port=4  SampleTime=1e-08
  wires:
  Selector/1 -> d_voltage_per_switching_state/1
  Selector1/1 -> q_voltage_per_switching_state/1
  Selector2/1 -> x_voltage_per_switching_state/1
  Selector3/1 -> y_voltage_per_switching_state/1
  multiplier_outbuff/1 -> Selector3/1, Selector2/1, Selector1/1, Selector/1
  Assignment/1 -> multiplier/2(In2)
  Assignment1/1 -> Assignment/1
  delayMatch4/1 -> Assignment1/1
  delayMatch6/1 -> multiplier1/2(In2)
  delayMatch5/1 -> multiplier2/2(In2)
  Selector6/1 -> Assignment2/2
  Assignment3/1 -> Assignment2/1
  adder/1 -> Selector9/2, Selector8/2, Selector7/2, Selector6/2, Selector5/2, Selector4/2
  t/1 -> Selector4/1
  t1/1 -> Selector5/1
  delayMatch3/1 -> multiplier3/2(In2)
  delayMatch2/1 -> multiplier4/2(In2)
  t2/1 -> Selector6/1
  Selector9/1 -> Assignment3/2
  const3/1 -> Assignment3/1
  const4/1 -> adder/2
  t3/1 -> Selector7/1
  t4/1 -> Selector8/1
  t5/1 -> Selector9/1
  const/1 -> t/1
  const1/1 -> t1/1
  const2/1 -> t2/1
  const5/1 -> t3/1
  const6/1 -> t4/1
  const7/1 -> t5/1
  delayMatch7/1 -> multiplier/1(In1)
  multiplier/1(Out1) -> multiplier_outbuff/1
  adder1/1(Out1) -> Assignment/2
  multiplier1/1(Out1) -> adder1/2(In2)
  multiplier2/1(Out1) -> adder1/1(In1)
  adder2/1(Out1) -> Assignment1/2
  uminus/1(Out1) -> multiplier2/1(In1)
  multiplier3/1(Out1) -> adder2/2(In2)
  multiplier4/1(Out1) -> adder2/1(In1)
  Assignment2/1 -> delayMatch/1
  t6/1 -> delayMatch1/1
  Selector8/1 -> delayMatch2/1
  Selector7/1 -> delayMatch3/1
  delayMatch/1 -> delayMatch4/1
  Selector5/1 -> delayMatch5/1
  Selector4/1 -> delayMatch6/1
  delayMatch1/1 -> delayMatch7/1
  sin_theta_el/1 -> multiplier3/1(In1), uminus/1(In1)
  cos_theta_el/1 -> multiplier4/1(In1), multiplier1/1(In1)
  u_dc_link_voltage/1 -> t6/4, t6/3, t6/2, t6/1
  Index/1 -> adder/1
